simulink model "straight_TMS3_noPH_ORC"  (R2022a)
settings: Solver=VariableStepAuto  StartTime=0.0  StopTime=3000  RelTol=1e-3
model workspace: external: MATLAB File parameters_straight.m (data not in the file)
undefined symbols (not defined in the file): BoP, cf, clch, clnt, const, h2o, htr, HX_ORC, ORC, pemel, prch
libraries: fl_lib x54, nesl_utility x19, SimscapeFluids_lib x5, slpidlib x3
(part 2 of 2)

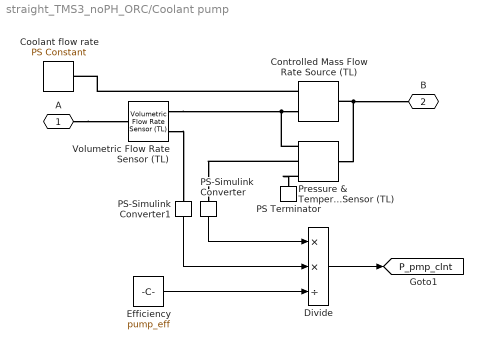
== system straight_TMS3_noPH_ORC/Coolant pump ==
  Controlled Mass Flow Rate Source (TL) : fl_lib/Thermal Liquid/Sources/Controlled Mass Flow Rate Source (TL)  area=clch.Ac_tot m^2
      settings: SourceProductBaseCode=PW,SS,VE  InternalSimscapePortConfiguration="{\"Bottom\":[],\"Left\":[{\"id\":\"A\",\"label\":\"A\",\"type\":\"foundation.thermal_liquid.thermal_liquid\"},{\"id\":\"M\",\"label\":\"M\",\"type\":\"input\"}],\"Right\":[{\"id\":\"B\",\"label\":\"B\",\"type\":\"foundation.thermal_liquid.thermal_liquid\"}],\"Top\":[]}"
  Coolant flow rate : fl_lib/Physical Signals/Sources/PS Constant  constant=clnt.mdot_stk*pemel.N_stk
      settings: SourceProductBaseCode=PW,SS,VE
  Divide : Product  Inputs=**/
  Efficiency : Constant  Value=pump_eff
  PS Terminator : fl_lib/Physical Signals/Sinks/PS Terminator
      settings: SourceProductBaseCode=PW,SS,VE
  PS-Simulink Converter : nesl_utility/PS-Simulink Converter  PhysicalDomain=network_engine_domain  SubClassName=ps_output  LeftPortType=input  RightPortType=output  PseudoPeriodic=off  Frequencies=[]  VectorFormat=inherit  Unit=Pa  AffineConversion=off
      settings: SourceProductBaseCode=SS,PW,VE
  PS-Simulink Converter1 : nesl_utility/PS-Simulink Converter  PhysicalDomain=network_engine_domain  SubClassName=ps_output  LeftPortType=input  RightPortType=output  PseudoPeriodic=off  Frequencies=[]  VectorFormat=inherit  Unit=m^3/s  AffineConversion=off
      settings: SourceProductBaseCode=SS,PW,VE
  Pressure & Temperature Sensor (TL) : fl_lib/Thermal Liquid/Sensors/Pressure & Temperature Sensor (TL)
      settings: SourceProductBaseCode=PW,SS,VE  InternalSimscapePortConfiguration="{\"Bottom\":[],\"Left\":[{\"id\":\"A\",\"label\":\"A\",\"type\":\"foundation.thermal_liquid.thermal_liquid\"}],\"Right\":[{\"id\":\"B\",\"label\":\"B\",\"type\":\"foundation.thermal_liquid.thermal_liquid\"},{\"id\":\"P\",\"label\":\"P\",\"type\":\"output\"},{\"id\":\"T\",\"label\":\"T\",\"type\":\"output\"}],\"Top\":[]}"
  Volumetric Flow Rate Sensor (TL) : fl_lib/Thermal Liquid/Sensors/Volumetric Flow Rate Sensor (TL)
      settings: SourceProductBaseCode=PW,SS,VE  InternalSimscapePortConfiguration="{\"Bottom\":[],\"Left\":[{\"id\":\"A\",\"label\":\"A\",\"type\":\"foundation.thermal_liquid.thermal_liquid\"}],\"Right\":[{\"id\":\"B\",\"label\":\"B\",\"type\":\"foundation.thermal_liquid.thermal_liquid\"},{\"id\":\"V\",\"label\":\"V\",\"type\":\"output\"}],\"Top\":[]}"
  A : PMIOPort  Side=Left
  B : PMIOPort  Port=2  Side=Right
  tag scope: P_pmp_clnt=global
  wires:
  Divide/1 -> [P_pmp_clnt]
  PS-Simulink Converter/1 -> Divide/1
  PS-Simulink Converter1/1 -> Divide/2
  Efficiency/1 -> Divide/3
  connections:
  Pressure & Temperature Sensor (TL)/RConn1 -- Volumetric Flow Rate Sensor (TL)/RConn1 -- Controlled Mass Flow Rate Source (TL)/LConn1
  Controlled Mass Flow Rate Source (TL)/RConn1 -- Pressure & Temperature Sensor (TL)/LConn1 -- B/RConn1
  Pressure & Temperature Sensor (TL)/RConn3 -- PS Terminator/LConn1
  Controlled Mass Flow Rate Source (TL)/LConn2 -- Coolant flow rate/RConn1
  A/RConn1 -- Volumetric Flow Rate Sensor (TL)/LConn1
  Volumetric Flow Rate Sensor (TL)/RConn2 -- PS-Simulink Converter1/LConn1
  Pressure & Temperature Sensor (TL)/RConn2 -- PS-Simulink Converter/LConn1

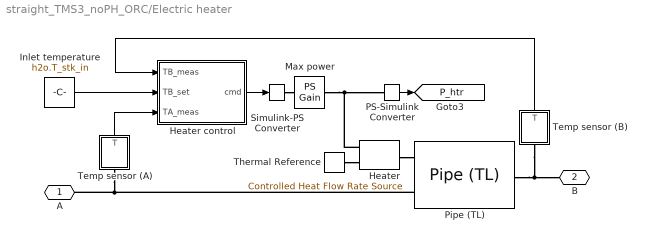
== system straight_TMS3_noPH_ORC/Electric heater ==
  Heater : fl_lib/Thermal/Thermal Sources/Controlled Heat Flow Rate Source
      settings: SourceProductBaseCode=PW,SS,VE
  Heater control : Subsystem
  Inlet temperature : Constant  Value=h2o.T_stk_in
  Max power : fl_lib/Physical Signals/Functions/PS Gain  gain=htr.PwrRt kW
      settings: SourceProductBaseCode=PW,SS,VE
  PS-Simulink Converter : nesl_utility/PS-Simulink Converter  PhysicalDomain=network_engine_domain  SubClassName=ps_output  LeftPortType=input  RightPortType=output  PseudoPeriodic=off  Frequencies=[]  VectorFormat=inherit  Unit=W  AffineConversion=off
      settings: SourceProductBaseCode=SS,PW,VE
  Pipe (TL) : fl_lib/Thermal Liquid/Elements/Pipe (TL)  length=htr.L m  area=prch.Ac_tot m^2  Dh=prch.D m  length_add=0.1*htr.L m  roughness=15e-6 m  Re_lam=2000  Re_tur=4000  shape_factor=64  Nu_lam=3.66  dynamic_compressibility=simscape.enum.onoff.off  inertia=simscape.enum.onoff.off  p0=0.101325 MPa  T0=amb.T_sea K  mdot0=0 kg/s
      settings: SourceProductBaseCode=PW,SS,VE
  Simulink-PS Converter : nesl_utility/Simulink-PS Converter  PhysicalDomain=network_engine_domain  SubClassName=ps_input  LeftPortType=input  RightPortType=output  PseudoPeriodic=off  Frequencies=[]  NoiseDistribution=none  NoiseParameters=[]  Unit=1  AffineConversion=off  FilteringAndDerivatives=provide  SimscapeFilterOrder=1  InputFilterTimeConstant=0.001  UdotUserProvided=0
      settings: SourceProductBaseCode=SS,PW,VE
  Temp sensor (A) : Subsystem
  Temp sensor (B) : Subsystem
  Thermal Reference : fl_lib/Thermal/Thermal Elements/Thermal Reference
      settings: SourceProductBaseCode=PW,SS,VE
  A : PMIOPort  Side=Right
  B : PMIOPort  Port=2  Side=Left
  tag scope: P_htr=global
  wires:
  Temp sensor (B)/1(T) -> Heater control/1(TB_meas)
  Temp sensor (A)/1(T) -> Heater control/3(TA_meas)
  Inlet temperature/1 -> Heater control/2(TB_set)
  Heater control/1(cmd) -> Simulink-PS Converter/1
  PS-Simulink Converter/1 -> [P_htr]
  connections:
  Pipe (TL)/LConn1 -- Temp sensor (A)/LConn1 -- A/RConn1
  Pipe (TL)/RConn1 -- B/RConn1 -- Temp sensor (B)/LConn1
  Heater/LConn1 -- Pipe (TL)/LConn2
  Thermal Reference/LConn1 -- Heater/RConn2
  Simulink-PS Converter/RConn1 -- Max power/LConn1
  Max power/RConn1 -- Heater/RConn1 -- PS-Simulink Converter/LConn1

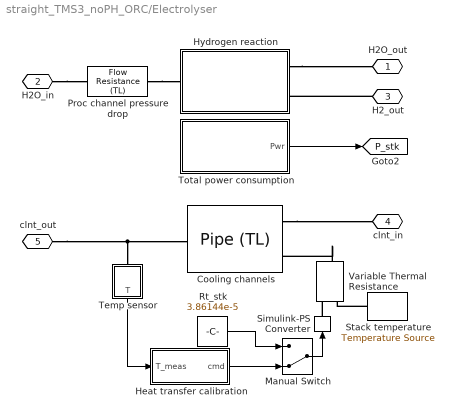
== system straight_TMS3_noPH_ORC/Electrolyser ==
  Cooling channels : SimscapeFluids_lib/Thermal Liquid/Pipes & Fittings/Pipe (TL)  dynamic_compressibility=simscape.enum.onoff.off  inertia=simscape.enum.onoff.off  num_segments=1  pipe_length=clch.L m  area=clch.Ac_tot m^2  wall_spec=fluids.thermal_liquid.pipes_fittings.enum.wall_spec.rigid  Dh=clch.Dh_stk m  wall_compliance=1.2e-6 m/MPa  wall_time_constant=0.01 s  elevation_spec=foundation.enum.constant_variable.constant  elevation_gain=0 m  g=9.81 m/s^2  pressure_loss_spec=fluids.thermal_liquid.pipes_fittings.enum.PressureLossSpec.Nominal  local_pressure_loss_spec=fluids.thermal_liquid.pipes_fittings.enum.LocalLossSpec.AggregateLength  length_add=1 m  loss_coefficient=0.1  roughness=15e-6 m  Re_friction_TLU=[400, 1000, 1500, 3000, 4000, 6000, 10000, 20000, 40000, 60000, 100000, 100000000]  friction_factor_TLU=[.264, .112, .071, .0417, .0387, .0268, .025, .0232, .0226, .022, .0214, .0214]  shape_factor=64  Re_lam=2300  Re_tur=3000  mdot_nominal=clnt.mdot_tot kg/s  p_diff_nominal=clnt.dp_stk Pa  mdot_threshold=1e-12 kg/s  heat_transfer_spec=fluids.thermal_liquid.pipes_fittings.enum.HeatTransferSpec.Gnielinski  mdot_nominal_heat=clnt.mdot_tot kg/s  T_in_nominal=clnt.T_stk_in K  T_out_nominal=clnt.T_stk_out K  p_in_nominal_heat=clnt.p_stk_in Pa  T_wall_nominal=pemel.T_stk K  a_coeff=0.023  b_Re_power=0.8  c_Pr_power=0.4  Nu_lam=3.66  Re_Colburn_TLU=[100, 150, 1000]  Colburn_factor_TLU=[.019, .013, .002]  Re_Nu_TLU=[100, 150, 1000]  Pr_Nu_TLU=[1, 10]  Nu_TLU=[3.72, 4.21; 3.75, 4.44; 4.21, 7.15]  T0_vec=amb.T K  p0_vec=0.101325 MPa  mdot0=0.1 kg/s
      settings: SourceProductBaseCode=SH
  Heat transfer calibration : Subsystem
  Hydrogen reaction : Subsystem
  Manual Switch : ManualSwitch  CurrentSetting=0
  Proc channel pressure drop : fl_lib/Thermal Liquid/Elements/Flow Resistance (TL)  delta_p_nominal=h2o.dp_stk bar  mdot_nominal=h2o.mdot_in_tot kg/s  area=prch.Ac_tot m^2  laminar_fraction=1e-3
      settings: SourceProductBaseCode=PW,SS,VE
  Rt_stk : Constant  Value=3.86144e-5
  Simulink-PS Converter : nesl_utility/Simulink-PS Converter  PhysicalDomain=network_engine_domain  SubClassName=ps_input  LeftPortType=input  RightPortType=output  PseudoPeriodic=off  Frequencies=[]  NoiseDistribution=none  NoiseParameters=[]  Unit=K/W  AffineConversion=off  FilteringAndDerivatives=provide  SimscapeFilterOrder=1  InputFilterTimeConstant=0.001  UdotUserProvided=0
      settings: SourceProductBaseCode=SS,PW,VE
  Stack temperature : fl_lib/Thermal/Thermal Sources/Temperature Source  temperature=pemel.T_stk K
      settings: SourceProductBaseCode=PW,SS,VE
  Temp sensor : Subsystem
  Total power consumption : Subsystem
  Variable Thermal Resistance : fl_lib/Thermal/Thermal Elements/Variable Thermal Resistance  R_min=0 K/W  T_specify=off  T_priority=None  T=0 K  T_nominal_specify=off  T_nominal_unit=K  T_nominal_value=1  Q_specify=off  Q_priority=None  Q=0 W  Q_nominal_specify=off  Q_nominal_unit=W  Q_nominal_value=1
      settings: SourceProductBaseCode=PW,SS,VE  InternalSimscapePortConfiguration="{\"Bottom\":[],\"Left\":[{\"id\":\"A\",\"label\":\"A\",\"type\":\"foundation.thermal.thermal\"},{\"id\":\"R\",\"label\":\"R\",\"type\":\"input\"}],\"Right\":[{\"id\":\"B\",\"label\":\"B\",\"type\":\"foundation.thermal.thermal\"}],\"Top\":[]}"
  H2O_out : PMIOPort  Side=Left
  H2O_in : PMIOPort  Port=2  Side=Left
  H2_out : PMIOPort  Port=3  Side=Right
  clnt_in : PMIOPort  Port=4  Side=Right
  clnt_out : PMIOPort  Port=5  Side=Left
  tag scope: P_stk=global
  wires:
  Total power consumption/1(Pwr) -> [P_stk]
  Manual Switch/1 -> Simulink-PS Converter/1
  Temp sensor/1(T) -> Heat transfer calibration/1(T_meas)
  Heat transfer calibration/1(cmd) -> Manual Switch/2
  Rt_stk/1 -> Manual Switch/1
  connections:
  clnt_out/RConn1 -- Cooling channels/RConn1 -- Temp sensor/LConn1
  Cooling channels/LConn1 -- clnt_in/RConn1
  Stack temperature/LConn1 -- Variable Thermal Resistance/LConn1
  Variable Thermal Resistance/RConn1 -- Cooling channels/LConn2
  H2_out/RConn1 -- Hydrogen reaction/RConn2
  H2O_in/RConn1 -- Proc channel pressure drop/LConn1
  Hydrogen reaction/RConn1 -- H2O_out/RConn1
  Simulink-PS Converter/RConn1 -- Variable Thermal Resistance/LConn2
  Proc channel pressure drop/RConn1 -- Hydrogen reaction/LConn1

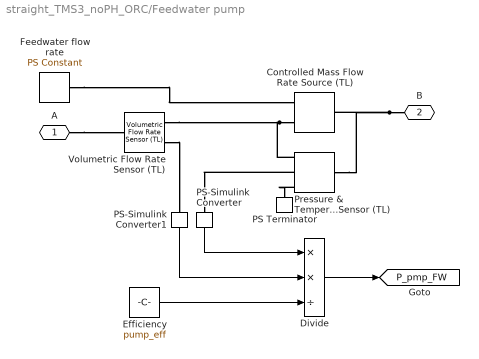
== system straight_TMS3_noPH_ORC/Feedwater pump ==
  Controlled Mass Flow Rate Source (TL) : fl_lib/Thermal Liquid/Sources/Controlled Mass Flow Rate Source (TL)  area=prch.Ac_tot m^2
      settings: SourceProductBaseCode=PW,SS,VE  InternalSimscapePortConfiguration="{\"Bottom\":[],\"Left\":[{\"id\":\"A\",\"label\":\"A\",\"type\":\"foundation.thermal_liquid.thermal_liquid\"},{\"id\":\"M\",\"label\":\"M\",\"type\":\"input\"}],\"Right\":[{\"id\":\"B\",\"label\":\"B\",\"type\":\"foundation.thermal_liquid.thermal_liquid\"}],\"Top\":[]}"
  Divide : Product  Inputs=**/
  Efficiency : Constant  Value=pump_eff
  Feedwater flow rate : fl_lib/Physical Signals/Sources/PS Constant  constant=h2o.mdot_in_tot kg/s
      settings: SourceProductBaseCode=PW,SS,VE
  PS Terminator : fl_lib/Physical Signals/Sinks/PS Terminator
      settings: SourceProductBaseCode=PW,SS,VE
  PS-Simulink Converter : nesl_utility/PS-Simulink Converter  PhysicalDomain=network_engine_domain  SubClassName=ps_output  LeftPortType=input  RightPortType=output  PseudoPeriodic=off  Frequencies=[]  VectorFormat=inherit  Unit=Pa  AffineConversion=off
      settings: SourceProductBaseCode=SS,PW,VE
  PS-Simulink Converter1 : nesl_utility/PS-Simulink Converter  PhysicalDomain=network_engine_domain  SubClassName=ps_output  LeftPortType=input  RightPortType=output  PseudoPeriodic=off  Frequencies=[]  VectorFormat=inherit  Unit=m^3/s  AffineConversion=off
      settings: SourceProductBaseCode=SS,PW,VE
  Pressure & Temperature Sensor (TL) : fl_lib/Thermal Liquid/Sensors/Pressure & Temperature Sensor (TL)
      settings: SourceProductBaseCode=PW,SS,VE  InternalSimscapePortConfiguration="{\"Bottom\":[],\"Left\":[{\"id\":\"A\",\"label\":\"A\",\"type\":\"foundation.thermal_liquid.thermal_liquid\"}],\"Right\":[{\"id\":\"B\",\"label\":\"B\",\"type\":\"foundation.thermal_liquid.thermal_liquid\"},{\"id\":\"P\",\"label\":\"P\",\"type\":\"output\"},{\"id\":\"T\",\"label\":\"T\",\"type\":\"output\"}],\"Top\":[]}"
  Volumetric Flow Rate Sensor (TL) : fl_lib/Thermal Liquid/Sensors/Volumetric Flow Rate Sensor (TL)
      settings: SourceProductBaseCode=PW,SS,VE  InternalSimscapePortConfiguration="{\"Bottom\":[],\"Left\":[{\"id\":\"A\",\"label\":\"A\",\"type\":\"foundation.thermal_liquid.thermal_liquid\"}],\"Right\":[{\"id\":\"B\",\"label\":\"B\",\"type\":\"foundation.thermal_liquid.thermal_liquid\"},{\"id\":\"V\",\"label\":\"V\",\"type\":\"output\"}],\"Top\":[]}"
  A : PMIOPort  Side=Left
  B : PMIOPort  Port=2  Side=Right
  tag scope: P_pmp_FW=global
  wires:
  Efficiency/1 -> Divide/3
  PS-Simulink Converter1/1 -> Divide/2
  PS-Simulink Converter/1 -> Divide/1
  Divide/1 -> [P_pmp_FW]
  connections:
  Pressure & Temperature Sensor (TL)/RConn2 -- PS-Simulink Converter/LConn1
  Volumetric Flow Rate Sensor (TL)/RConn2 -- PS-Simulink Converter1/LConn1
  A/RConn1 -- Volumetric Flow Rate Sensor (TL)/LConn1
  Feedwater flow rate/RConn1 -- Controlled Mass Flow Rate Source (TL)/LConn2
  Pressure & Temperature Sensor (TL)/RConn3 -- PS Terminator/LConn1
  B/RConn1 -- Controlled Mass Flow Rate Source (TL)/RConn1 -- Pressure & Temperature Sensor (TL)/LConn1
  Controlled Mass Flow Rate Source (TL)/LConn1 -- Volumetric Flow Rate Sensor (TL)/RConn1 -- Pressure & Temperature Sensor (TL)/RConn1

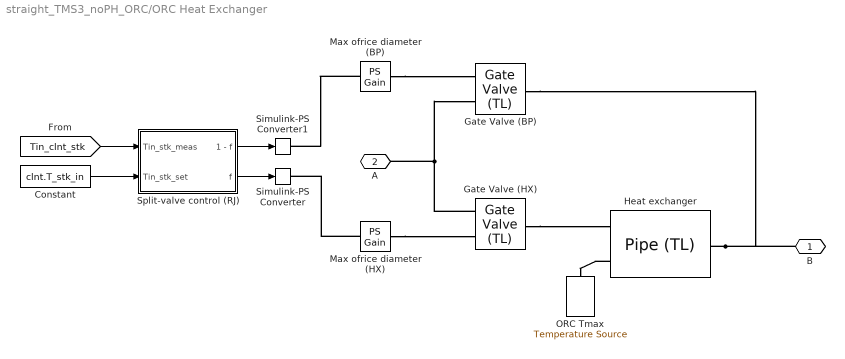
== system straight_TMS3_noPH_ORC/ORC Heat Exchanger ==
  Constant : Constant  Value=clnt.T_stk_in
  Gate Valve (BP) : SimscapeFluids_lib/Thermal Liquid/Valves & Orifices/Flow Control Valves/Gate Valve (TL)  diam_orifice=0.9*clch.D m  S_min=0 m  area_leak=1e-12 m^2  smoothing_factor=0.01  area=clch.Ac_tot m^2  Cd=0.9  Re_c=4000
      settings: SourceProductBaseCode=SH  InternalSimscapePortConfiguration="{\"Bottom\":[],\"Left\":[{\"id\":\"A\",\"label\":\"A\",\"type\":\"foundation.thermal_liquid.thermal_liquid\"},{\"id\":\"S\",\"label\":\"S\",\"type\":\"input\"}],\"Right\":[{\"id\":\"B\",\"label\":\"B\",\"type\":\"foundation.thermal_liquid.thermal_liquid\"}],\"Top\":[]}"
  Gate Valve (HX) : SimscapeFluids_lib/Thermal Liquid/Valves & Orifices/Flow Control Valves/Gate Valve (TL)  diam_orifice=0.9*clch.D m  S_min=0 m  area_leak=1e-12 m^2  smoothing_factor=0.01  area=clch.Ac_tot m^2  Cd=0.9  Re_c=4000
      settings: SourceProductBaseCode=SH  InternalSimscapePortConfiguration="{\"Bottom\":[],\"Left\":[{\"id\":\"A\",\"label\":\"A\",\"type\":\"foundation.thermal_liquid.thermal_liquid\"},{\"id\":\"S\",\"label\":\"S\",\"type\":\"input\"}],\"Right\":[{\"id\":\"B\",\"label\":\"B\",\"type\":\"foundation.thermal_liquid.thermal_liquid\"}],\"Top\":[]}"
  Heat exchanger : fl_lib/Thermal Liquid/Elements/Pipe (TL)  length=cf.L_rjORC*HX_ORC.L_h m  area=clch.Ac_tot m^2  Dh=clch.D m  length_add=0.1*HX_ORC.L_h m  roughness=15e-6 m  Re_lam=2300  Re_tur=3000  shape_factor=64  Nu_lam=3.66  dynamic_compressibility=simscape.enum.onoff.off  inertia=simscape.enum.onoff.off  p0=0.101325 MPa  T0=amb.T K  mdot0=0 kg/s
      settings: SourceProductBaseCode=PW,SS,VE
  Max ofrice diameter (BP) : fl_lib/Physical Signals/Functions/PS Gain  gain=clch.D m
      settings: SourceProductBaseCode=PW,SS,VE
  Max ofrice diameter (HX) : fl_lib/Physical Signals/Functions/PS Gain  gain=clch.D m
      settings: SourceProductBaseCode=PW,SS,VE
  ORC Tmax : fl_lib/Thermal/Thermal Sources/Temperature Source  temperature=ORC.Tmax K
      settings: SourceProductBaseCode=PW,SS,VE
  Simulink-PS Converter : nesl_utility/Simulink-PS Converter  PhysicalDomain=network_engine_domain  SubClassName=ps_input  LeftPortType=input  RightPortType=output  PseudoPeriodic=off  Frequencies=[]  NoiseDistribution=none  NoiseParameters=[]  Unit=1  AffineConversion=off  FilteringAndDerivatives=provide  SimscapeFilterOrder=1  InputFilterTimeConstant=0.001  UdotUserProvided=0
      settings: SourceProductBaseCode=SS,PW,VE
  Simulink-PS Converter1 : nesl_utility/Simulink-PS Converter  PhysicalDomain=network_engine_domain  SubClassName=ps_input  LeftPortType=input  RightPortType=output  PseudoPeriodic=off  Frequencies=[]  NoiseDistribution=none  NoiseParameters=[]  Unit=1  AffineConversion=off  FilteringAndDerivatives=provide  SimscapeFilterOrder=1  InputFilterTimeConstant=0.001  UdotUserProvided=0
      settings: SourceProductBaseCode=SS,PW,VE
  Split-valve control (RJ) : Subsystem
  B : PMIOPort  Side=Left
  A : PMIOPort  Port=2  Side=Right
  wires:
  Split-valve control (RJ)/2(f) -> Simulink-PS Converter/1
  Split-valve control (RJ)/1(1 - f) -> Simulink-PS Converter1/1
  [Tin_clnt_stk] -> Split-valve control (RJ)/1(Tin_stk_meas)
  Constant/1 -> Split-valve control (RJ)/2(Tin_stk_set)
  connections:
  Gate Valve (HX)/RConn1 -- Heat exchanger/LConn1
  Gate Valve (HX)/LConn1 -- Gate Valve (BP)/LConn1 -- A/RConn1
  Heat exchanger/RConn1 -- Gate Valve (BP)/RConn1 -- B/RConn1
  Max ofrice diameter (BP)/LConn1 -- Simulink-PS Converter1/RConn1
  Max ofrice diameter (BP)/RConn1 -- Gate Valve (BP)/LConn2
  Max ofrice diameter (HX)/LConn1 -- Simulink-PS Converter/RConn1
  Max ofrice diameter (HX)/RConn1 -- Gate Valve (HX)/LConn2
  Heat exchanger/LConn2 -- ORC Tmax/LConn1

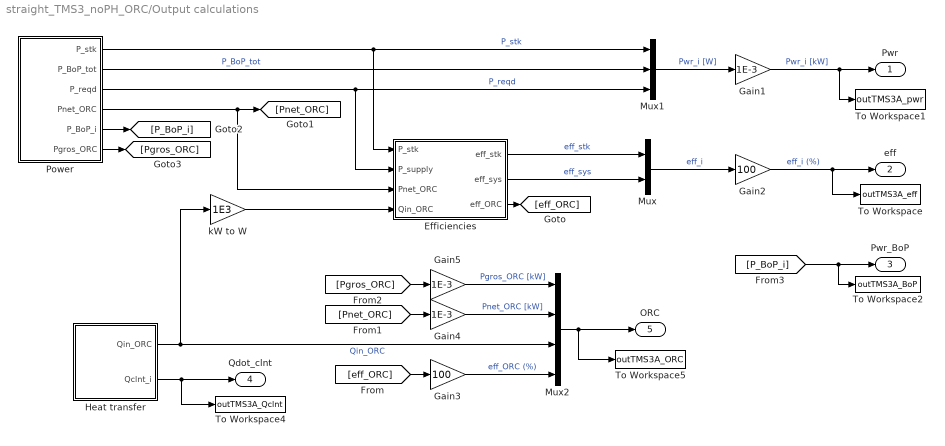
== system straight_TMS3_noPH_ORC/Output calculations ==
  Efficiencies : Subsystem
  Gain1 : Gain  Gain=1E-3
  Gain2 : Gain  Gain=100
  Gain3 : Gain  Gain=100
  Gain4 : Gain  Gain=1E-3
  Gain5 : Gain  Gain=1E-3
  Heat transfer : Subsystem
  Mux : Mux  Inputs=2
  Mux1 : Mux  Inputs=3
  Mux2 : Mux
  Power : Subsystem
  To Workspace : ToWorkspace  VariableName=outTMS3A_eff  SampleTime=-1
      settings: MaxDataPoints=1  Save2DSignal=2-D array (concatenate along first dimension)
  To Workspace1 : ToWorkspace  VariableName=outTMS3A_pwr  SampleTime=-1
      settings: MaxDataPoints=1  Save2DSignal=2-D array (concatenate along first dimension)
  To Workspace2 : ToWorkspace  VariableName=outTMS3A_BoP  SampleTime=-1
      settings: MaxDataPoints=1  Save2DSignal=2-D array (concatenate along first dimension)
  To Workspace4 : ToWorkspace  VariableName=outTMS3A_Qclnt  SampleTime=-1
      settings: MaxDataPoints=1  Save2DSignal=2-D array (concatenate along first dimension)
  To Workspace5 : ToWorkspace  VariableName=outTMS3A_ORC  SampleTime=-1
      settings: MaxDataPoints=1  Save2DSignal=2-D array (concatenate along first dimension)
  kW to W : Gain  Gain=1E3
  Pwr : Outport
  eff : Outport  Port=2
  Pwr_BoP : Outport  Port=3
  Qdot_clnt : Outport  Port=4
  ORC : Outport  Port=5
  wires:
  Gain2/1 -> eff/1, To Workspace/1  "eff_i (%)"
  Power/1(P_stk) -> Efficiencies/1(P_stk), Mux1/1  "P_stk"
  Power/3(P_reqd) -> Efficiencies/2(P_supply), Mux1/3  "P_reqd"
  Power/2(P_BoP_tot) -> Mux1/2  "P_BoP_tot"
  Mux1/1 -> Gain1/1  "Pwr_i [W]"
  Heat transfer/2(Qclnt_i) -> To Workspace4/1, Qdot_clnt/1
  Gain1/1 -> To Workspace1/1, Pwr/1  "Pwr_i [kW]"
  Power/4(Pnet_ORC) -> Efficiencies/3(Pnet_ORC), [Pnet_ORC]
  Heat transfer/1(Qin_ORC) -> Mux2/3, kW to W/1  "Qin_ORC"
  Gain3/1 -> Mux2/4  "eff_ORC (%)"
  Mux2/1 -> ORC/1, To Workspace5/1
  Gain4/1 -> Mux2/2  "Pnet_ORC [kW]"
  Gain5/1 -> Mux2/1  "Pgros_ORC [kW]"
  kW to W/1 -> Efficiencies/4(Qin_ORC)
  [eff_ORC] -> Gain3/1
  [Pnet_ORC] -> Gain4/1
  Power/5(P_BoP_i) -> [P_BoP_i]
  Power/6(Pgros_ORC) -> [Pgros_ORC]
  [Pgros_ORC] -> Gain5/1
  [P_BoP_i] -> To Workspace2/1, Pwr_BoP/1
  Efficiencies/1(eff_stk) -> Mux/1  "eff_stk"
  Efficiencies/3(eff_ORC) -> [eff_ORC]
  Mux/1 -> Gain2/1  "eff_i"
  Efficiencies/2(eff_sys) -> Mux/2  "eff_sys"

== system straight_TMS3_noPH_ORC/Q sensor (rj_out) ==
  Mass & Energy Flow Rate Sensor (TL) : fl_lib/Thermal Liquid/Sensors/Mass & Energy Flow Rate Sensor (TL)
      settings: SourceProductBaseCode=PW,SS,VE  InternalSimscapePortConfiguration="{\"Bottom\":[],\"Left\":[{\"id\":\"A\",\"label\":\"A\",\"type\":\"foundation.thermal_liquid.thermal_liquid\"}],\"Right\":[{\"id\":\"B\",\"label\":\"B\",\"type\":\"foundation.thermal_liquid.thermal_liquid\"},{\"id\":\"M\",\"label\":\"M\",\"type\":\"output\"},{\"id\":\"PHI\",\"label\":\"Phi\",\"type\":\"output\"}],\"Top\":[]}"
  PS Terminator : fl_lib/Physical Signals/Sinks/PS Terminator
      settings: SourceProductBaseCode=PW,SS,VE
  PS-Simulink Converter2 : nesl_utility/PS-Simulink Converter  PhysicalDomain=network_engine_domain  SubClassName=ps_output  LeftPortType=input  RightPortType=output  PseudoPeriodic=off  Frequencies=[]  VectorFormat=1-D array  Unit=kW  AffineConversion=off
      settings: SourceProductBaseCode=SS,PW,VE
  B : PMIOPort  Side=Right
  A : PMIOPort  Port=2  Side=Left
  tag scope: Phi_clnt_rjOut=global
  wires:
  PS-Simulink Converter2/1 -> [Phi_clnt_rjOut]
  connections:
  PS Terminator/LConn1 -- Mass & Energy Flow Rate Sensor (TL)/RConn2
  Mass & Energy Flow Rate Sensor (TL)/RConn3 -- PS-Simulink Converter2/LConn1
  Mass & Energy Flow Rate Sensor (TL)/RConn1 -- B/RConn1
  Mass & Energy Flow Rate Sensor (TL)/LConn1 -- A/RConn1

== system straight_TMS3_noPH_ORC/Q sensor (stk_in) ==
  Mass & Energy Flow Rate Sensor (TL) : fl_lib/Thermal Liquid/Sensors/Mass & Energy Flow Rate Sensor (TL)
      settings: SourceProductBaseCode=PW,SS,VE  InternalSimscapePortConfiguration="{\"Bottom\":[],\"Left\":[{\"id\":\"A\",\"label\":\"A\",\"type\":\"foundation.thermal_liquid.thermal_liquid\"}],\"Right\":[{\"id\":\"B\",\"label\":\"B\",\"type\":\"foundation.thermal_liquid.thermal_liquid\"},{\"id\":\"M\",\"label\":\"M\",\"type\":\"output\"},{\"id\":\"PHI\",\"label\":\"Phi\",\"type\":\"output\"}],\"Top\":[]}"
  PS Terminator : fl_lib/Physical Signals/Sinks/PS Terminator
      settings: SourceProductBaseCode=PW,SS,VE
  PS-Simulink Converter2 : nesl_utility/PS-Simulink Converter  PhysicalDomain=network_engine_domain  SubClassName=ps_output  LeftPortType=input  RightPortType=output  PseudoPeriodic=off  Frequencies=[]  VectorFormat=1-D array  Unit=kW  AffineConversion=off
      settings: SourceProductBaseCode=SS,PW,VE
  B : PMIOPort  Side=Right
  A : PMIOPort  Port=2  Side=Left
  tag scope: Phi_clnt_stkIn=global
  wires:
  PS-Simulink Converter2/1 -> [Phi_clnt_stkIn]
  connections:
  Mass & Energy Flow Rate Sensor (TL)/LConn1 -- A/RConn1
  Mass & Energy Flow Rate Sensor (TL)/RConn1 -- B/RConn1
  Mass & Energy Flow Rate Sensor (TL)/RConn3 -- PS-Simulink Converter2/LConn1
  PS Terminator/LConn1 -- Mass & Energy Flow Rate Sensor (TL)/RConn2

== system straight_TMS3_noPH_ORC/Q sensor (stk_out) ==
  Mass & Energy Flow Rate Sensor (TL) : fl_lib/Thermal Liquid/Sensors/Mass & Energy Flow Rate Sensor (TL)
      settings: SourceProductBaseCode=PW,SS,VE  InternalSimscapePortConfiguration="{\"Bottom\":[],\"Left\":[{\"id\":\"A\",\"label\":\"A\",\"type\":\"foundation.thermal_liquid.thermal_liquid\"}],\"Right\":[{\"id\":\"B\",\"label\":\"B\",\"type\":\"foundation.thermal_liquid.thermal_liquid\"},{\"id\":\"M\",\"label\":\"M\",\"type\":\"output\"},{\"id\":\"PHI\",\"label\":\"Phi\",\"type\":\"output\"}],\"Top\":[]}"
  PS Terminator : fl_lib/Physical Signals/Sinks/PS Terminator
      settings: SourceProductBaseCode=PW,SS,VE
  PS-Simulink Converter2 : nesl_utility/PS-Simulink Converter  PhysicalDomain=network_engine_domain  SubClassName=ps_output  LeftPortType=input  RightPortType=output  PseudoPeriodic=off  Frequencies=[]  VectorFormat=1-D array  Unit=kW  AffineConversion=off
      settings: SourceProductBaseCode=SS,PW,VE
  B : PMIOPort  Side=Right
  A : PMIOPort  Port=2  Side=Left
  tag scope: Phi_clnt_stkOut=global
  wires:
  PS-Simulink Converter2/1 -> [Phi_clnt_stkOut]
  connections:
  PS Terminator/LConn1 -- Mass & Energy Flow Rate Sensor (TL)/RConn2
  Mass & Energy Flow Rate Sensor (TL)/RConn3 -- PS-Simulink Converter2/LConn1
  Mass & Energy Flow Rate Sensor (TL)/RConn1 -- B/RConn1
  Mass & Energy Flow Rate Sensor (TL)/LConn1 -- A/RConn1

== system straight_TMS3_noPH_ORC/T sensor ==
  Absolute Reference (TL)2 : fl_lib/Thermal Liquid/Elements/Absolute Reference (TL)
      settings: SourceProductBaseCode=PW,SS,VE
  PS-Simulink Converter4 : nesl_utility/PS-Simulink Converter  PhysicalDomain=network_engine_domain  SubClassName=ps_output  LeftPortType=input  RightPortType=output  PseudoPeriodic=off  Frequencies=[]  VectorFormat=1-D array  Unit=K  AffineConversion=off
      settings: SourceProductBaseCode=SS,PW,VE
  Pressure & Temperature Sensor (TL)2 : fl_lib/Thermal Liquid/Sensors/Pressure & Temperature Sensor (TL)
      settings: SourceProductBaseCode=PW,SS,VE  InternalSimscapePortConfiguration="{\"Bottom\":[],\"Left\":[{\"id\":\"A\",\"label\":\"A\",\"type\":\"foundation.thermal_liquid.thermal_liquid\"}],\"Right\":[{\"id\":\"B\",\"label\":\"B\",\"type\":\"foundation.thermal_liquid.thermal_liquid\"},{\"id\":\"P\",\"label\":\"P\",\"type\":\"output\"},{\"id\":\"T\",\"label\":\"T\",\"type\":\"output\"}],\"Top\":[]}"
  A : PMIOPort  Side=Left
  tag scope: Tin_clnt_stk=global
  wires:
  PS-Simulink Converter4/1 -> [Tin_clnt_stk]
  connections:
  Pressure & Temperature Sensor (TL)2/LConn1 -- A/RConn1
  Pressure & Temperature Sensor (TL)2/RConn3 -- PS-Simulink Converter4/LConn1
  Pressure & Temperature Sensor (TL)2/RConn1 -- Absolute Reference (TL)2/LConn1

== system straight_TMS3_noPH_ORC/mdot sensor ==
  Mass & Energy Flow Rate Sensor (G) : fl_lib/Gas/Sensors/Mass & Energy Flow Rate Sensor (G)
      settings: SourceProductBaseCode=PW,SS,VE  InternalSimscapePortConfiguration="{\"Bottom\":[],\"Left\":[{\"id\":\"A\",\"label\":\"A\",\"type\":\"foundation.gas.gas\"}],\"Right\":[{\"id\":\"B\",\"label\":\"B\",\"type\":\"foundation.gas.gas\"},{\"id\":\"M\",\"label\":\"M\",\"type\":\"output\"},{\"id\":\"PHI\",\"label\":\"Phi\",\"type\":\"output\"}],\"Top\":[]}"
  PS Terminator : fl_lib/Physical Signals/Sinks/PS Terminator
      settings: SourceProductBaseCode=PW,SS,VE
  PS-Simulink Converter2 : nesl_utility/PS-Simulink Converter  PhysicalDomain=network_engine_domain  SubClassName=ps_output  LeftPortType=input  RightPortType=output  PseudoPeriodic=off  Frequencies=[]  VectorFormat=1-D array  Unit=kg/s  AffineConversion=off
      settings: SourceProductBaseCode=SS,PW,VE
  B : PMIOPort  Side=Right
  A : PMIOPort  Port=2  Side=Left
  tag scope: mdot_h2=global
  wires:
  PS-Simulink Converter2/1 -> [mdot_h2]
  connections:
  Mass & Energy Flow Rate Sensor (G)/RConn1 -- B/RConn1
  Mass & Energy Flow Rate Sensor (G)/RConn2 -- PS-Simulink Converter2/LConn1
  Mass & Energy Flow Rate Sensor (G)/LConn1 -- A/RConn1
  Mass & Energy Flow Rate Sensor (G)/RConn3 -- PS Terminator/LConn1

== system straight_TMS3_noPH_ORC/Electric heater/Heater control ==
  TB_meas : Inport
  TB_set : Inport  Port=2
  TA_meas : Inport  Port=3
  Constant : Constant  Value=0
  Delay : TransferFcn  Denominator=[1 1]
  Don't heat if already at stack inlet temp : Switch  Threshold=h2o.T_stk_in  SaturateOnIntegerOverflow=off  InputSameDT=off
  PID Controller : slpidlib/PID Controller  Controller=PID  Form=Ideal  TimeDomain=Continuous-time  UseExternalTs=off  SampleTime=-1  IntegratorMethod=Forward Euler  FilterMethod=Forward Euler  ControllerParametersSource=internal  P=22.0976847072654  I=0.0930858056504815  UseKiTs=off  D=1.11880828545236  N=1378.56209413945  UseFilter=on  TunerSelectOption=Transfer Function Based (PID Tuner App)  InitialConditionSource=internal  InitialConditionForIntegrator=0  InitialConditionForFilter=0  DifferentiatorICPrevScaledInput=0  ExternalReset=none  TrackingMode=off  Kt=1  LimitOutput=on  SatLimitsSource=internal  UpperSaturationLimit=1  LowerSaturationLimit=0  LinearizeAsGain=on  AntiWindupMode=back-calculation  Kb=0.1  POutMin=[]  POutMax=[]  IOutMin=[]  IOutMax=[]  DOutMin=[]  DOutMax=[]  NOutMin=[]  NOutMax=[]  SumOutMin=[]  SumOutMax=[]  SaturationOutMin=[]  SaturationOutMax=[]  PParamMin=[]  PParamMax=[]  IParamMin=[]  IParamMax=[]  DParamMin=[]  DParamMax=[]  NParamMin=[]  NParamMax=[]  KbParamMin=[]  KbParamMax=[]  KtParamMin=[]  KtParamMax=[]  KbOutMin=[]  KbOutMax=[]  KtOutMin=[]  KtOutMax=[]  IntegratorOutMin=[]  IntegratorOutMax=[]  FilterOutMin=[]  FilterOutMax=[]  SumI1OutMin=[]  SumI1OutMax=[]  SumI2OutMin=[]  SumI2OutMax=[]  SumI3OutMin=[]  SumI3OutMax=[]  SumI4OutMin=[]  SumI4OutMax=[]  SumDOutMin=[]  SumDOutMax=[]  DifferentiatorOutMin=[]  DifferentiatorOutMax=[]  FilterDiffOutCoefMin=[]  FilterDiffOutCoefMax=[]  ReciprocalOutMin=[]  ReciprocalOutMax=[]  SumDenOutMin=[]  SumDenOutMax=[]  SumNumOutMin=[]  SumNumOutMax=[]  DivideOutMin=[]  DivideOutMax=[]  UdiffTsProdOutMin=[]  UdiffTsProdOutMax=[]  NTsProdOutMin=[]  NTsProdOutMax=[]  UintegralTsProdOutMin=[]  UintegralTsProdOutMax=[]  UngainTsProdOutMin=[]  UngainTsProdOutMax=[]  IntegratorContinuousStateAttributes=''  IntegratorStateMustResolveToSignalObject=off  IntegratorRTWStateStorageClass=Auto  FilterContinuousStateAttributes=''  FilterStateMustResolveToSignalObject=off  FilterRTWStateStorageClass=Auto  ParallelPVariant=Passthrough  IdealPVariant=InternalParameters  IVariant=InternalParameters  DVariant=InternalParameters  IntegratorVariant=Continuous  SatVariant=Enabled  AWVariant=BackCalculation  PCopyVariant=Disabled  TRVariant=Disabled  FdbkBlocksVariant=Forward  IdealPFdbkVariant=Disabled  SatFdbkVariant=Disabled  DerivativeFilterVariant=ContFilter  NVariant=InternalParameters  NCopyVariant=Disabled  FilterICVariant=InternalICsFilter  IntegratorICVariant=InternalICs  ExternalResetVariant=Disabled  TRSumVariant=Passthrough  SumFdbkVariant=Disabled  SumVariant=Sum_PID  TsampFilterVariant=InternalTs  TsampNgainVariant=Passthrough  TsampIntegralVariant=Passthrough  ExternalSaturationOutDataTypeStr=Inherit: Same as second input  aMode=0
  Sum : Sum  Inputs=|+-
  cmd : Outport
  wires:
  TA_meas/1 -> Don't heat if already at stack inlet temp/2
  Constant/1 -> Don't heat if already at stack inlet temp/1
  Don't heat if already at stack inlet temp/1 -> Delay/1
  TB_meas/1 -> Sum/2
  TB_set/1 -> Sum/1
  Sum/1 -> PID Controller/1
  PID Controller/1 -> Don't heat if already at stack inlet temp/3
  Delay/1 -> cmd/1

== system straight_TMS3_noPH_ORC/Electric heater/Temp sensor (A) ==
  Absolute Reference (TL)1 : fl_lib/Thermal Liquid/Elements/Absolute Reference (TL)
      settings: SourceProductBaseCode=PW,SS,VE
  PS Terminator1 : fl_lib/Physical Signals/Sinks/PS Terminator
      settings: SourceProductBaseCode=PW,SS,VE
  PS-Simulink Converter1 : nesl_utility/PS-Simulink Converter  PhysicalDomain=network_engine_domain  SubClassName=ps_output  LeftPortType=input  RightPortType=output  PseudoPeriodic=off  Frequencies=[]  VectorFormat=1-D array  Unit=K  AffineConversion=off
      settings: SourceProductBaseCode=SS,PW,VE
  Pressure & Temperature Sensor (TL)1 : fl_lib/Thermal Liquid/Sensors/Pressure & Temperature Sensor (TL)
      settings: SourceProductBaseCode=PW,SS,VE  InternalSimscapePortConfiguration="{\"Bottom\":[],\"Left\":[{\"id\":\"A\",\"label\":\"A\",\"type\":\"foundation.thermal_liquid.thermal_liquid\"}],\"Right\":[{\"id\":\"B\",\"label\":\"B\",\"type\":\"foundation.thermal_liquid.thermal_liquid\"},{\"id\":\"P\",\"label\":\"P\",\"type\":\"output\"},{\"id\":\"T\",\"label\":\"T\",\"type\":\"output\"}],\"Top\":[]}"
  A : PMIOPort  Side=Left
  T : Outport
  wires:
  PS-Simulink Converter1/1 -> T/1
  connections:
  Pressure & Temperature Sensor (TL)1/RConn3 -- PS-Simulink Converter1/LConn1
  Pressure & Temperature Sensor (TL)1/RConn2 -- PS Terminator1/LConn1
  Pressure & Temperature Sensor (TL)1/LConn1 -- A/RConn1
  Pressure & Temperature Sensor (TL)1/RConn1 -- Absolute Reference (TL)1/LConn1

== system straight_TMS3_noPH_ORC/Electric heater/Temp sensor (B) ==
  Absolute Reference (TL)1 : fl_lib/Thermal Liquid/Elements/Absolute Reference (TL)
      settings: SourceProductBaseCode=PW,SS,VE
  PS Terminator1 : fl_lib/Physical Signals/Sinks/PS Terminator
      settings: SourceProductBaseCode=PW,SS,VE
  PS-Simulink Converter1 : nesl_utility/PS-Simulink Converter  PhysicalDomain=network_engine_domain  SubClassName=ps_output  LeftPortType=input  RightPortType=output  PseudoPeriodic=off  Frequencies=[]  VectorFormat=1-D array  Unit=K  AffineConversion=off
      settings: SourceProductBaseCode=SS,PW,VE
  Pressure & Temperature Sensor (TL)1 : fl_lib/Thermal Liquid/Sensors/Pressure & Temperature Sensor (TL)
      settings: SourceProductBaseCode=PW,SS,VE  InternalSimscapePortConfiguration="{\"Bottom\":[],\"Left\":[{\"id\":\"A\",\"label\":\"A\",\"type\":\"foundation.thermal_liquid.thermal_liquid\"}],\"Right\":[{\"id\":\"B\",\"label\":\"B\",\"type\":\"foundation.thermal_liquid.thermal_liquid\"},{\"id\":\"P\",\"label\":\"P\",\"type\":\"output\"},{\"id\":\"T\",\"label\":\"T\",\"type\":\"output\"}],\"Top\":[]}"
  A : PMIOPort  Side=Left
  T : Outport
  wires:
  PS-Simulink Converter1/1 -> T/1
  connections:
  Pressure & Temperature Sensor (TL)1/RConn1 -- Absolute Reference (TL)1/LConn1
  Pressure & Temperature Sensor (TL)1/LConn1 -- A/RConn1
  Pressure & Temperature Sensor (TL)1/RConn2 -- PS Terminator1/LConn1
  Pressure & Temperature Sensor (TL)1/RConn3 -- PS-Simulink Converter1/LConn1

== system straight_TMS3_noPH_ORC/Electrolyser/Heat transfer calibration ==
  T_meas : Inport
  Constant : Constant  Value=clnt.T_stk_out
  Delay : TransferFcn  Denominator=[1 1]
  PID Controller : slpidlib/PID Controller  Controller=PID  Form=Ideal  TimeDomain=Continuous-time  UseExternalTs=off  SampleTime=-1  IntegratorMethod=Forward Euler  FilterMethod=Forward Euler  ControllerParametersSource=internal  P=-0.000189338981396971  I=0.784930022412218  UseKiTs=off  D=0.286068954623357  N=2759.12113964656  UseFilter=on  TunerSelectOption=Transfer Function Based (PID Tuner App)  InitialConditionSource=internal  InitialConditionForIntegrator=0  InitialConditionForFilter=0  DifferentiatorICPrevScaledInput=0  ExternalReset=none  TrackingMode=off  Kt=1  LimitOutput=off  SatLimitsSource=internal  UpperSaturationLimit=inf  LowerSaturationLimit=0  LinearizeAsGain=on  AntiWindupMode=back-calculation  Kb=0.1  POutMin=[]  POutMax=[]  IOutMin=[]  IOutMax=[]  DOutMin=[]  DOutMax=[]  NOutMin=[]  NOutMax=[]  SumOutMin=[]  SumOutMax=[]  SaturationOutMin=[]  SaturationOutMax=[]  PParamMin=[]  PParamMax=[]  IParamMin=[]  IParamMax=[]  DParamMin=[]  DParamMax=[]  NParamMin=[]  NParamMax=[]  KbParamMin=[]  KbParamMax=[]  KtParamMin=[]  KtParamMax=[]  KbOutMin=[]  KbOutMax=[]  KtOutMin=[]  KtOutMax=[]  IntegratorOutMin=[]  IntegratorOutMax=[]  FilterOutMin=[]  FilterOutMax=[]  SumI1OutMin=[]  SumI1OutMax=[]  SumI2OutMin=[]  SumI2OutMax=[]  SumI3OutMin=[]  SumI3OutMax=[]  SumI4OutMin=[]  SumI4OutMax=[]  SumDOutMin=[]  SumDOutMax=[]  DifferentiatorOutMin=[]  DifferentiatorOutMax=[]  FilterDiffOutCoefMin=[]  FilterDiffOutCoefMax=[]  ReciprocalOutMin=[]  ReciprocalOutMax=[]  SumDenOutMin=[]  SumDenOutMax=[]  SumNumOutMin=[]  SumNumOutMax=[]  DivideOutMin=[]  DivideOutMax=[]  UdiffTsProdOutMin=[]  UdiffTsProdOutMax=[]  NTsProdOutMin=[]  NTsProdOutMax=[]  UintegralTsProdOutMin=[]  UintegralTsProdOutMax=[]  UngainTsProdOutMin=[]  UngainTsProdOutMax=[]  IntegratorContinuousStateAttributes=''  IntegratorStateMustResolveToSignalObject=off  IntegratorRTWStateStorageClass=Auto  FilterContinuousStateAttributes=''  FilterStateMustResolveToSignalObject=off  FilterRTWStateStorageClass=Auto  ParallelPVariant=Passthrough  IdealPVariant=InternalParameters  IVariant=InternalParameters  DVariant=InternalParameters  IntegratorVariant=Continuous  SatVariant=Disabled  AWVariant=Passthrough  PCopyVariant=Disabled  TRVariant=Disabled  FdbkBlocksVariant=Forward  IdealPFdbkVariant=Disabled  SatFdbkVariant=Disabled  DerivativeFilterVariant=ContFilter  NVariant=InternalParameters  NCopyVariant=Disabled  FilterICVariant=InternalICsFilter  IntegratorICVariant=InternalICs  ExternalResetVariant=Disabled  TRSumVariant=Passthrough  SumFdbkVariant=Disabled  SumVariant=Sum_PID  TsampFilterVariant=InternalTs  TsampNgainVariant=Passthrough  TsampIntegralVariant=Passthrough  ExternalSaturationOutDataTypeStr=Inherit: Same as second input  aMode=0
  Sum : Sum  Inputs=|+-
  cmd : Outport
  wires:
  PID Controller/1 -> Delay/1
  T_meas/1 -> Sum/2
  Constant/1 -> Sum/1
  Sum/1 -> PID Controller/1
  Delay/1 -> cmd/1

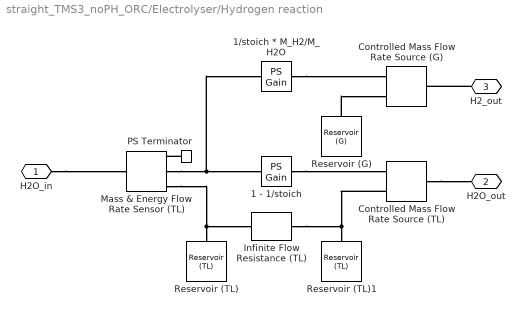
== system straight_TMS3_noPH_ORC/Electrolyser/Hydrogen reaction ==
  1 - 1/stoich : fl_lib/Physical Signals/Functions/PS Gain  gain=1 - (1/h2o.stoich)
      settings: SourceProductBaseCode=PW,SS,VE
  1/stoich * M_H2/M_H2O : fl_lib/Physical Signals/Functions/PS Gain  gain=(1/h2o.stoich)*(const.M_h2/const.M_h2o)
      settings: SourceProductBaseCode=PW,SS,VE
  Controlled Mass Flow Rate Source (G) : fl_lib/Gas/Sources/Controlled Mass Flow Rate Source (G)  power_spec=foundation.enum.power_spec.none  area_A=prch.Ac_tot m^2  area_B=prch.Ac_tot m^2
      settings: SourceProductBaseCode=PW,SS,VE  InternalSimscapePortConfiguration="{\"Bottom\":[],\"Left\":[{\"id\":\"A\",\"label\":\"A\",\"type\":\"foundation.gas.gas\"},{\"id\":\"M\",\"label\":\"M\",\"type\":\"input\"}],\"Right\":[{\"id\":\"B\",\"label\":\"B\",\"type\":\"foundation.gas.gas\"}],\"Top\":[]}"
  Controlled Mass Flow Rate Source (TL) : fl_lib/Thermal Liquid/Sources/Controlled Mass Flow Rate Source (TL)  area=prch.Ac_tot m^2
      settings: SourceProductBaseCode=PW,SS,VE  InternalSimscapePortConfiguration="{\"Bottom\":[],\"Left\":[{\"id\":\"A\",\"label\":\"A\",\"type\":\"foundation.thermal_liquid.thermal_liquid\"},{\"id\":\"M\",\"label\":\"M\",\"type\":\"input\"}],\"Right\":[{\"id\":\"B\",\"label\":\"B\",\"type\":\"foundation.thermal_liquid.thermal_liquid\"}],\"Top\":[]}"
  Infinite Flow Resistance (TL) : fl_lib/Thermal Liquid/Elements/Infinite Flow Resistance (TL)  p_specify=on  p_priority=None  p=0 MPa  p_nominal_specify=off  p_nominal_unit=MPa  p_nominal_value=1  T_specify=off  T_priority=None  T=0 K  T_nominal_specify=off  T_nominal_unit=K  T_nominal_value=1
      settings: SourceProductBaseCode=PW,SS,VE  InternalSimscapePortConfiguration="{\"Bottom\":[],\"Left\":[{\"id\":\"A\",\"label\":\"A\",\"type\":\"foundation.thermal_liquid.thermal_liquid\"}],\"Right\":[{\"id\":\"B\",\"label\":\"B\",\"type\":\"foundation.thermal_liquid.thermal_liquid\"}],\"Top\":[]}"
  Mass & Energy Flow Rate Sensor (TL) : fl_lib/Thermal Liquid/Sensors/Mass & Energy Flow Rate Sensor (TL)
      settings: SourceProductBaseCode=PW,SS,VE  InternalSimscapePortConfiguration="{\"Bottom\":[],\"Left\":[{\"id\":\"A\",\"label\":\"A\",\"type\":\"foundation.thermal_liquid.thermal_liquid\"}],\"Right\":[{\"id\":\"B\",\"label\":\"B\",\"type\":\"foundation.thermal_liquid.thermal_liquid\"},{\"id\":\"M\",\"label\":\"M\",\"type\":\"output\"},{\"id\":\"PHI\",\"label\":\"Phi\",\"type\":\"output\"}],\"Top\":[]}"
  PS Terminator : fl_lib/Physical Signals/Sinks/PS Terminator
      settings: SourceProductBaseCode=PW,SS,VE
  Reservoir (G) : fl_lib/Gas/Elements/Reservoir (G)  pressure_spec=foundation.enum.pressure_spec.specified  reservoir_pressure=pemel.p_ca Pa  reservoir_temperature=pemel.T_stk K  area_A=prch.Ac_tot m^2
      settings: SourceProductBaseCode=PW,SS,VE
  Reservoir (TL) : fl_lib/Thermal Liquid/Elements/Reservoir (TL)  pressure_spec=foundation.enum.pressure_spec.atmospheric  reservoir_pressure=0.101325 MPa  reservoir_temperature=h2o.T_stk_in K  area=prch.Ac_tot m^2
      settings: SourceProductBaseCode=PW,SS,VE
  Reservoir (TL)1 : fl_lib/Thermal Liquid/Elements/Reservoir (TL)  pressure_spec=foundation.enum.pressure_spec.atmospheric  reservoir_pressure=0.101325 MPa  reservoir_temperature=h2o.T_stk_out K  area=prch.Ac_tot m^2
      settings: SourceProductBaseCode=PW,SS,VE
  H2O_in : PMIOPort  Side=Left
  H2O_out : PMIOPort  Port=2  Side=Right
  H2_out : PMIOPort  Port=3  Side=Right
  connections:
  Mass & Energy Flow Rate Sensor (TL)/RConn2 -- 1/stoich * M_H2/M_H2O/LConn1 -- 1 - 1/stoich/LConn1
  Controlled Mass Flow Rate Source (TL)/LConn1 -- Infinite Flow Resistance (TL)/RConn1 -- Reservoir (TL)1/LConn1
  1 - 1/stoich/RConn1 -- Controlled Mass Flow Rate Source (TL)/LConn2
  Mass & Energy Flow Rate Sensor (TL)/RConn1 -- Infinite Flow Resistance (TL)/LConn1 -- Reservoir (TL)/LConn1
  Reservoir (G)/LConn1 -- Controlled Mass Flow Rate Source (G)/LConn1
  Controlled Mass Flow Rate Source (TL)/RConn1 -- H2O_out/RConn1
  PS Terminator/LConn1 -- Mass & Energy Flow Rate Sensor (TL)/RConn3
  1/stoich * M_H2/M_H2O/RConn1 -- Controlled Mass Flow Rate Source (G)/LConn2
  H2_out/RConn1 -- Controlled Mass Flow Rate Source (G)/RConn1
  H2O_in/RConn1 -- Mass & Energy Flow Rate Sensor (TL)/LConn1

== system straight_TMS3_noPH_ORC/Electrolyser/Temp sensor ==
  Absolute Reference (TL)1 : fl_lib/Thermal Liquid/Elements/Absolute Reference (TL)
      settings: SourceProductBaseCode=PW,SS,VE
  PS Terminator1 : fl_lib/Physical Signals/Sinks/PS Terminator
      settings: SourceProductBaseCode=PW,SS,VE
  PS-Simulink Converter1 : nesl_utility/PS-Simulink Converter  PhysicalDomain=network_engine_domain  SubClassName=ps_output  LeftPortType=input  RightPortType=output  PseudoPeriodic=off  Frequencies=[]  VectorFormat=1-D array  Unit=K  AffineConversion=off
      settings: SourceProductBaseCode=SS,PW,VE
  Pressure & Temperature Sensor (TL)1 : fl_lib/Thermal Liquid/Sensors/Pressure & Temperature Sensor (TL)
      settings: SourceProductBaseCode=PW,SS,VE  InternalSimscapePortConfiguration="{\"Bottom\":[],\"Left\":[{\"id\":\"A\",\"label\":\"A\",\"type\":\"foundation.thermal_liquid.thermal_liquid\"}],\"Right\":[{\"id\":\"B\",\"label\":\"B\",\"type\":\"foundation.thermal_liquid.thermal_liquid\"},{\"id\":\"P\",\"label\":\"P\",\"type\":\"output\"},{\"id\":\"T\",\"label\":\"T\",\"type\":\"output\"}],\"Top\":[]}"
  A : PMIOPort  Side=Left
  T : Outport
  wires:
  PS-Simulink Converter1/1 -> T/1
  connections:
  Pressure & Temperature Sensor (TL)1/RConn3 -- PS-Simulink Converter1/LConn1
  Pressure & Temperature Sensor (TL)1/RConn2 -- PS Terminator1/LConn1
  Pressure & Temperature Sensor (TL)1/LConn1 -- A/RConn1
  Pressure & Temperature Sensor (TL)1/RConn1 -- Absolute Reference (TL)1/LConn1

== system straight_TMS3_noPH_ORC/Electrolyser/Total power consumption ==
  I : Constant  Value=pemel.I
  N_stk : Constant  Value=pemel.N_stk
  Product : Product  Inputs=3
  V_stk : Constant  Value=pemel.V_stk
  Pwr : Outport
  wires:
  I/1 -> Product/3
  V_stk/1 -> Product/2
  N_stk/1 -> Product/1
  Product/1 -> Pwr/1

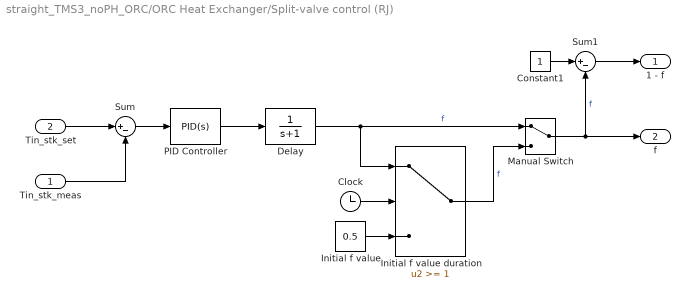
== system straight_TMS3_noPH_ORC/ORC Heat Exchanger/Split-valve control (RJ) ==
  Tin_stk_meas : Inport
  Tin_stk_set : Inport  Port=2
  Clock : Clock
  Constant1 : Constant
  Delay : TransferFcn  Denominator=[1 1]
  Initial f value : Constant  Value=0.5
  Initial f value duration : Switch  Threshold=1  SaturateOnIntegerOverflow=off  InputSameDT=off
  Manual Switch : ManualSwitch
  PID Controller : slpidlib/PID Controller  Controller=PID  Form=Ideal  TimeDomain=Continuous-time  UseExternalTs=off  SampleTime=-1  IntegratorMethod=Forward Euler  FilterMethod=Forward Euler  ControllerParametersSource=internal  P=-0.555708182490552  I=0.95717123634426  UseKiTs=off  D=0.096496205335411  N=3.15255555770467  UseFilter=on  TunerSelectOption=Transfer Function Based (PID Tuner App)  InitialConditionSource=internal  InitialConditionForIntegrator=0  InitialConditionForFilter=0  DifferentiatorICPrevScaledInput=0  ExternalReset=none  TrackingMode=off  Kt=1  LimitOutput=on  SatLimitsSource=internal  UpperSaturationLimit=1  LowerSaturationLimit=0  LinearizeAsGain=on  AntiWindupMode=back-calculation  Kb=0.1  POutMin=[]  POutMax=[]  IOutMin=[]  IOutMax=[]  DOutMin=[]  DOutMax=[]  NOutMin=[]  NOutMax=[]  SumOutMin=[]  SumOutMax=[]  SaturationOutMin=[]  SaturationOutMax=[]  PParamMin=[]  PParamMax=[]  IParamMin=[]  IParamMax=[]  DParamMin=[]  DParamMax=[]  NParamMin=[]  NParamMax=[]  KbParamMin=[]  KbParamMax=[]  KtParamMin=[]  KtParamMax=[]  KbOutMin=[]  KbOutMax=[]  KtOutMin=[]  KtOutMax=[]  IntegratorOutMin=[]  IntegratorOutMax=[]  FilterOutMin=[]  FilterOutMax=[]  SumI1OutMin=[]  SumI1OutMax=[]  SumI2OutMin=[]  SumI2OutMax=[]  SumI3OutMin=[]  SumI3OutMax=[]  SumI4OutMin=[]  SumI4OutMax=[]  SumDOutMin=[]  SumDOutMax=[]  DifferentiatorOutMin=[]  DifferentiatorOutMax=[]  FilterDiffOutCoefMin=[]  FilterDiffOutCoefMax=[]  ReciprocalOutMin=[]  ReciprocalOutMax=[]  SumDenOutMin=[]  SumDenOutMax=[]  SumNumOutMin=[]  SumNumOutMax=[]  DivideOutMin=[]  DivideOutMax=[]  UdiffTsProdOutMin=[]  UdiffTsProdOutMax=[]  NTsProdOutMin=[]  NTsProdOutMax=[]  UintegralTsProdOutMin=[]  UintegralTsProdOutMax=[]  UngainTsProdOutMin=[]  UngainTsProdOutMax=[]  IntegratorContinuousStateAttributes=''  IntegratorStateMustResolveToSignalObject=off  IntegratorRTWStateStorageClass=Auto  FilterContinuousStateAttributes=''  FilterStateMustResolveToSignalObject=off  FilterRTWStateStorageClass=Auto  ParallelPVariant=Passthrough  IdealPVariant=InternalParameters  IVariant=InternalParameters  DVariant=InternalParameters  IntegratorVariant=Continuous  SatVariant=Enabled  AWVariant=BackCalculation  PCopyVariant=Disabled  TRVariant=Disabled  FdbkBlocksVariant=Forward  IdealPFdbkVariant=Disabled  SatFdbkVariant=Disabled  DerivativeFilterVariant=ContFilter  NVariant=InternalParameters  NCopyVariant=Disabled  FilterICVariant=InternalICsFilter  IntegratorICVariant=InternalICs  ExternalResetVariant=Disabled  TRSumVariant=Passthrough  SumFdbkVariant=Disabled  SumVariant=Sum_PID  TsampFilterVariant=InternalTs  TsampNgainVariant=Passthrough  TsampIntegralVariant=Passthrough  ExternalSaturationOutDataTypeStr=Inherit: Same as second input  aMode=0
  Sum : Sum  Inputs=|+-
  Sum1 : Sum  Inputs=|+-
  1 - f : Outport
  f : Outport  Port=2
  wires:
  Sum1/1 -> 1 - f/1
  Sum/1 -> PID Controller/1
  Tin_stk_set/1 -> Sum/1
  Tin_stk_meas/1 -> Sum/2
  PID Controller/1 -> Delay/1
  Constant1/1 -> Sum1/1
  Initial f value/1 -> Initial f value duration/3
  Clock/1 -> Initial f value duration/2
  Delay/1 -> Initial f value duration/1, Manual Switch/1  "f"
  Initial f value duration/1 -> Manual Switch/2  "f"
  Manual Switch/1 -> Sum1/2, f/1  "f"

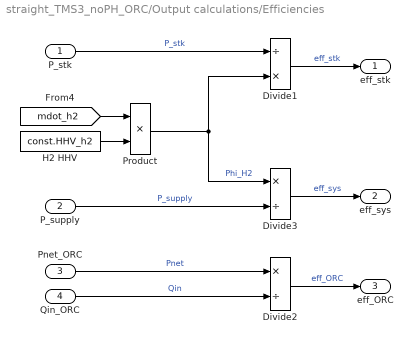
== system straight_TMS3_noPH_ORC/Output calculations/Efficiencies ==
  P_stk : Inport
  P_supply : Inport  Port=2
  Pnet_ORC : Inport  Port=3
  Qin_ORC : Inport  Port=4
  Divide1 : Product  Inputs=/*
  Divide2 : Product  Inputs=*/
  Divide3 : Product  Inputs=*/
  H2 HHV : Constant  Value=const.HHV_h2
  Product : Product
  eff_stk : Outport
  eff_sys : Outport  Port=2
  eff_ORC : Outport  Port=3
  wires:
  Pnet_ORC/1 -> Divide2/1  "Pnet"
  Qin_ORC/1 -> Divide2/2  "Qin"
  Divide2/1 -> eff_ORC/1  "eff_ORC"
  [mdot_h2] -> Product/1
  Divide1/1 -> eff_stk/1  "eff_stk"
  Divide3/1 -> eff_sys/1  "eff_sys"
  P_stk/1 -> Divide1/1  "P_stk"
  H2 HHV/1 -> Product/2
  Product/1 -> Divide1/2, Divide3/1  "Phi_H2"
  P_supply/1 -> Divide3/2  "P_supply"

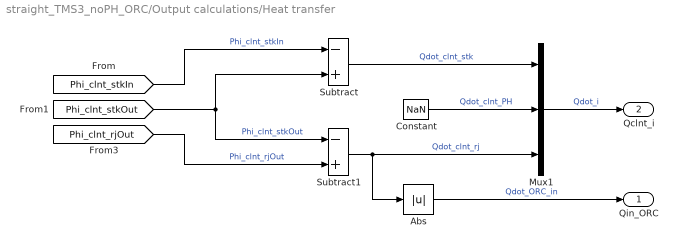
== system straight_TMS3_noPH_ORC/Output calculations/Heat transfer ==
  Abs : Abs  SaturateOnIntegerOverflow=off
  Constant : Constant  Value=NaN
  Mux1 : Mux  Inputs=3
  Subtract : Sum  Inputs=-+
  Subtract1 : Sum  Inputs=-+
  Qin_ORC : Outport
  Qclnt_i : Outport  Port=2
  wires:
  Abs/1 -> Qin_ORC/1  "Qdot_ORC_in"
  [Phi_clnt_stkOut] -> Subtract1/1, Subtract/2  "Phi_clnt_stkOut"
  Mux1/1 -> Qclnt_i/1  "Qdot_i"
  Constant/1 -> Mux1/2  "Qdot_clnt_PH"
  [Phi_clnt_stkIn] -> Subtract/1  "Phi_clnt_stkIn"
  Subtract1/1 -> Abs/1, Mux1/3  "Qdot_clnt_rj"
  [Phi_clnt_rjOut] -> Subtract1/2  "Phi_clnt_rjOut"
  Subtract/1 -> Mux1/1  "Qdot_clnt_stk"

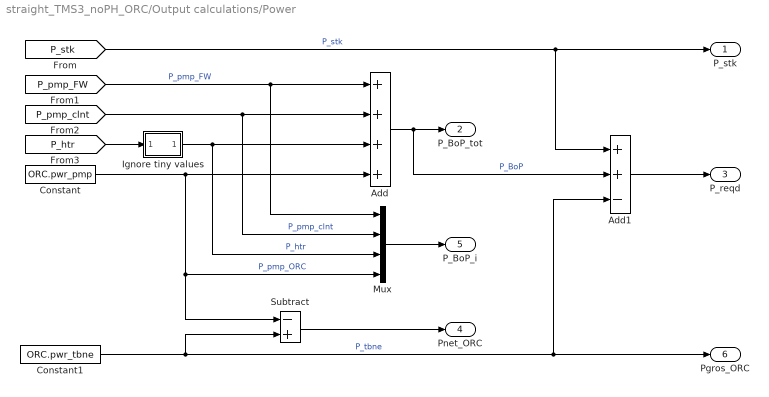
== system straight_TMS3_noPH_ORC/Output calculations/Power ==
  Add : Sum  Inputs=++++
  Add1 : Sum  Inputs=++-
  Constant : Constant  Value=ORC.pwr_pmp
  Constant1 : Constant  Value=ORC.pwr_tbne
  Ignore tiny values : Subsystem
  Mux : Mux
  Subtract : Sum  Inputs=-+
  P_stk : Outport
  P_BoP_tot : Outport  Port=2
  P_reqd : Outport  Port=3
  Pnet_ORC : Outport  Port=4
  P_BoP_i : Outport  Port=5
  Pgros_ORC : Outport  Port=6
  wires:
  [P_stk] -> P_stk/1, Add1/1  "P_stk"
  Add/1 -> Add1/2, P_BoP_tot/1  "P_BoP"
  Mux/1 -> P_BoP_i/1
  Add1/1 -> P_reqd/1
  Constant1/1 -> Pgros_ORC/1, Add1/3, Subtract/2  "P_tbne"
  [P_pmp_FW] -> Mux/1, Add/1  "P_pmp_FW"
  [P_pmp_clnt] -> Mux/2, Add/2  "P_pmp_clnt"
  Constant/1 -> Add/4, Subtract/1, Mux/4  "P_pmp_ORC"
  Subtract/1 -> Pnet_ORC/1
  [P_htr] -> Ignore tiny values/1(In1)
  Ignore tiny values/1(Out1) -> Add/3, Mux/3  "P_htr"

== system straight_TMS3_noPH_ORC/Output calculations/Power/Ignore tiny values ==
  In1 : Inport
  Constant2 : Constant  Value=0
  Switch : Switch  Threshold=0.1  SaturateOnIntegerOverflow=off  InputSameDT=off
  Out1 : Outport
  wires:
  In1/1 -> Switch/2, Switch/1
  Constant2/1 -> Switch/3
  Switch/1 -> Out1/1  "P_htr"
